simulink model "lab6"  (R2019b)
settings: Solver=VariableStepAuto  StartTime=0.0  StopTime=10.0  RelTol=1e-3
settings Model: Creator=Michał  LastModifiedBy=Michał

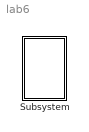
== system lab6 ==
  Subsystem : Subsystem  mask{h1=4, h2=2, Swy1=0.2, Swy2=0.2, S1=1, S2=1, Qwe=2, g=9.81, phi1=1, phi2=1}

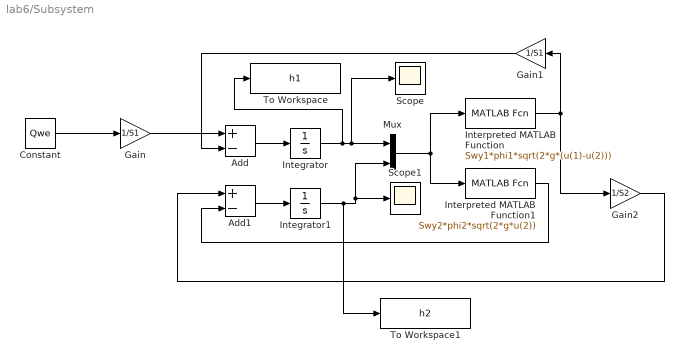
== system lab6/Subsystem ==
  Add : Sum  Inputs=+-
  Add1 : Sum  Inputs=+-
  Constant : Constant  Value=Qwe
  Gain : Gain  Gain=1/S1
  Gain1 : Gain  Gain=1/S1
  Gain2 : Gain  Gain=1/S2
  Integrator : Integrator  InitialCondition=h1
  Integrator1 : Integrator  InitialCondition=h2
  Interpreted MATLAB Function : MATLABFcn  MATLABFcn=Swy1*phi1*sqrt(2*g*(u(1)-u(2)))
  Interpreted MATLAB Function1 : MATLABFcn  MATLABFcn=Swy2*phi2*sqrt(2*g*u(2))
  Mux : Mux  Inputs=2
  Scope : Scope
  Scope1 : Scope
  To Workspace : ToWorkspace  VariableName=h1  SaveFormat=Timeseries  SampleTime=-1
  To Workspace1 : ToWorkspace  VariableName=h2  SaveFormat=Timeseries  SampleTime=-1
  wires:
  Add1/1 -> Integrator1/1
  Gain/1 -> Add/1
  Gain1/1 -> Add/2
  Mux/1 -> Interpreted MATLAB Function1/1, Interpreted MATLAB Function/1
  Integrator/1 -> To Workspace/1, Scope/1, Mux/1
  Interpreted MATLAB Function1/1 -> Add1/2
  Add/1 -> Integrator/1
  Integrator1/1 -> To Workspace1/1, Scope1/1, Mux/2
  Interpreted MATLAB Function/1 -> Gain1/1, Gain2/1
  Gain2/1 -> Add1/1
  Constant/1 -> Gain/1
